simulink model "RBFNN_1221"  (R2018a)
settings: Solver=FixedStepAuto  StartTime=0.0  StopTime=inf  FixedStep=0.001  RelTol=1e-3  EnableMultiTasking=on
undefined symbols (not defined in the file): HIL, j, qc_get_step_size
libraries: dsparch4 x28, quarc_library x17, simulink x7, vrlib x1
(part 2 of 6)

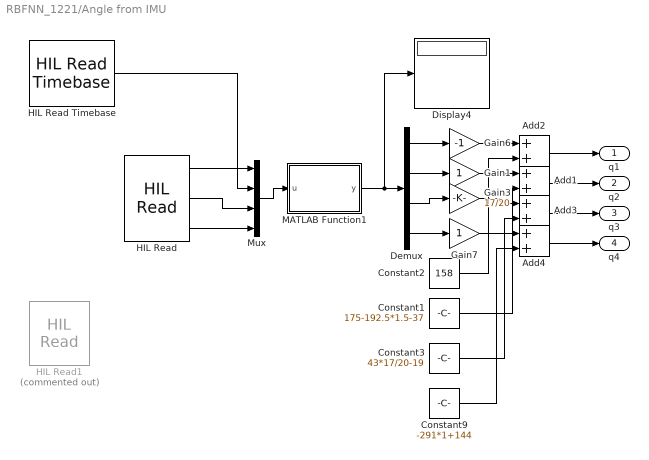
== system RBFNN_1221/Angle from IMU ==
  Add{1..4} (4 alike) : Sum
  Constant1 : Constant  Value=175-192.5*1.5-37
  Constant2 : Constant  Value=158
  Constant3 : Constant  Value=43*17/20-19
  Constant9 : Constant  Value=-291*1+144
  Demux : Demux
  Display4 : Display
  Gain1 : Gain
  Gain3 : Gain  Gain=17/20
  Gain6 : Gain  Gain=-1
  Gain7 : Gain
  HIL Read : quarc_library/Data Acquisition/Generic/Immediate I//O/HIL Read  object_name=HIL-1  analog_channels=[1 4 7]  encoder_channels=[]  digital_channels=[]  other_channels=[]  sample_time=qc_get_step_size  active=on  vector_output=off  data_type_mode=Inherit via back propagation  encoder_data_type=double  digital_data_type=boolean
  HIL Read Timebase : quarc_library/Data Acquisition/Generic/Timebases/HIL Read Timebase  object_name=HIL-2  clock=0  analog_channels=0  encoder_channels=[]  digital_channels=[]  other_channels=[]  samples_in_buffer=max(ceil(1/qc_get_step_size), 1)  active=on  vector_output=off  data_type_mode=Inherit via back propagation  encoder_data_type=double  digital_data_type=boolean
  HIL Read1 : quarc_library/Data Acquisition/Generic/Immediate I//O/HIL Read  Commented=on  object_name=HIL-2  analog_channels=[0]  encoder_channels=[]  digital_channels=[]  other_channels=[]  sample_time=qc_get_step_size  active=on  vector_output=off  data_type_mode=Inherit via back propagation  encoder_data_type=double  digital_data_type=boolean
  MATLAB Function1 : MATLAB Function  TreatAsAtomicUnit=on
  Mux : Mux
  q1 : Outport
  q2 : Outport  Port=2
  "q3 " : Outport  Port=3
  q4 : Outport  Port=4
  wires:
  Constant2/1 -> Add2/2
  Gain6/1 -> Add2/1
  Add2/1 -> q1/1
  Mux/1 -> MATLAB Function1/1(u)
  MATLAB Function1/1(y) -> Display4/1, Demux/1
  Demux/1 -> Gain6/1
  Gain3/1 -> Add3/1
  Gain7/1 -> Add4/1
  Constant3/1 -> Add3/2
  Constant9/1 -> Add4/2
  Add3/1 -> "q3 "/1
  Add4/1 -> q4/1
  HIL Read/1 -> Mux/1
  HIL Read/2 -> Mux/3
  HIL Read/3 -> Mux/4
  Demux/3 -> Gain3/1
  Demux/4 -> Gain7/1
  Demux/2 -> Gain1/1
  Gain1/1 -> Add1/1
  Constant1/1 -> Add1/2
  Add1/1 -> q2/1
  HIL Read Timebase/1 -> Mux/2

== system RBFNN_1221/Nan Switch ==
  control input : Inport
  angle signal : Inport  Port=2
  Constant4 : Constant  Value=0
  Mux : Mux
  Switch : Switch
  control : Outport
  wires:
  Switch/1 -> control/1
  control input/1 -> Switch/1
  angle signal/1 -> Switch/2
  Constant4/1 -> Mux/1, Mux/2, Mux/3, Mux/4
  Mux/1 -> Switch/3

== system RBFNN_1221/P1 ==
  Analog Filter Design1 : dsparch4/Analog Filter Design  method=Butterworth  filttype=Lowpass  N=2  Wlo=0.9  Whi=80  Rp=2  Rs=40
  Analog Filter Design2 : dsparch4/Analog Filter Design  method=Butterworth  filttype=Lowpass  N=2  Wlo=0.9  Whi=80  Rp=2  Rs=40
  HIL Read Analog : quarc_library/Data Acquisition/Generic/Immediate I//O/HIL Read Analog  object_name=HIL-1  channels=[2:3]  sample_time=qc_get_step_size  active=on  vector_output=off
  Manual Switch : ManualSwitch  CurrentSetting=0
  Manual Switch1 : ManualSwitch  CurrentSetting=0
  pin : Outport
  pout : Outport  Port=2
  wires:
  Manual Switch1/1 -> pout/1
  Manual Switch/1 -> pin/1
  HIL Read Analog/1 -> Analog Filter Design2/1, Manual Switch/1
  HIL Read Analog/2 -> Analog Filter Design1/1, Manual Switch1/1
  Analog Filter Design2/1 -> Manual Switch/2
  Analog Filter Design1/1 -> Manual Switch1/2

== system RBFNN_1221/P2 ==
  Analog Filter Design1 : dsparch4/Analog Filter Design  method=Butterworth  filttype=Lowpass  N=2  Wlo=0.9  Whi=80  Rp=2  Rs=40
  Analog Filter Design2 : dsparch4/Analog Filter Design  method=Butterworth  filttype=Lowpass  N=2  Wlo=0.9  Whi=80  Rp=2  Rs=40
  Demux : Demux  Outputs=2
  HIL Read Analog : quarc_library/Data Acquisition/Generic/Immediate I//O/HIL Read Analog  object_name=HIL-2  channels=[2:3]  sample_time=qc_get_step_size  active=on  vector_output=off
  Manual Switch : ManualSwitch
  Mux : Mux  Inputs=2
  Mux1 : Mux  Inputs=2
  pout : Outport
  pin : Outport  Port=2
  wires:
  HIL Read Analog/2 -> Analog Filter Design1/1
  HIL Read Analog/1 -> Analog Filter Design2/1
  Manual Switch/1 -> Demux/1
  Demux/1 -> pin/1
  Mux1/1 -> Manual Switch/2
  Mux/1 -> Manual Switch/1
  Analog Filter Design1/1 -> Mux1/1, Mux/2
  Demux/2 -> pout/1
  Analog Filter Design2/1 -> Mux1/2, Mux/1

== system RBFNN_1221/P3 ==
  Analog Filter Design1 : dsparch4/Analog Filter Design  method=Butterworth  filttype=Lowpass  N=2  Wlo=0.9  Whi=80  Rp=2  Rs=40
  Analog Filter Design2 : dsparch4/Analog Filter Design  method=Butterworth  filttype=Lowpass  N=2  Wlo=0.9  Whi=80  Rp=2  Rs=40
  HIL Read Analog : quarc_library/Data Acquisition/Generic/Immediate I//O/HIL Read Analog  object_name=HIL-1  channels=[5:6]  sample_time=qc_get_step_size  active=on  vector_output=off
  Scope : Scope  NumInputPorts=2
  pin : Outport
  pout : Outport  Port=2
  wires:
  Analog Filter Design1/1 -> pout/1
  Analog Filter Design2/1 -> pin/1
  HIL Read Analog/2 -> Scope/2, Analog Filter Design1/1
  HIL Read Analog/1 -> Scope/1, Analog Filter Design2/1

== system RBFNN_1221/P4 ==
  Analog Filter Design1 : dsparch4/Analog Filter Design  method=Butterworth  filttype=Lowpass  N=2  Wlo=0.9  Whi=80  Rp=2  Rs=40
  Analog Filter Design2 : dsparch4/Analog Filter Design  method=Butterworth  filttype=Lowpass  N=2  Wlo=0.9  Whi=80  Rp=2  Rs=40
  Demux : Demux  Outputs=2
  HIL Read Analog : quarc_library/Data Acquisition/Generic/Immediate I//O/HIL Read Analog  object_name=HIL-2  channels=[6:7]  sample_time=qc_get_step_size  active=on  vector_output=off
  Manual Switch : ManualSwitch
  Mux : Mux  Inputs=2
  Mux1 : Mux  Inputs=2
  pin : Outport
  pout : Outport  Port=2
  wires:
  HIL Read Analog/2 -> Analog Filter Design1/1
  HIL Read Analog/1 -> Analog Filter Design2/1
  Analog Filter Design2/1 -> Mux1/2, Mux/1
  Analog Filter Design1/1 -> Mux1/1, Mux/2
  Mux/1 -> Manual Switch/1
  Manual Switch/1 -> Demux/1
  Demux/1 -> pin/1
  Demux/2 -> pout/1
  Mux1/1 -> Manual Switch/2

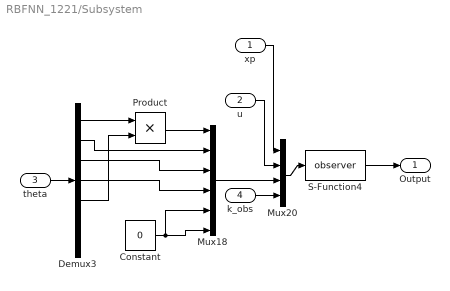
== system RBFNN_1221/Subsystem ==
  xp : Inport
  u : Inport  Port=2
  theta : Inport  Port=3
  k_obs : Inport  Port=4
  Constant : Constant  Value=0
  Demux3 : Demux  Outputs=7
  Mux18 : Mux  Inputs=6
  Mux20 : Mux
  Product : Product
  S-Function4 : S-Function  FunctionName=observer  SFunctionDeploymentMode=off  EnableBusSupport=off
  Output : Outport
  wires:
  theta/1 -> Demux3/1
  Demux3/1 -> Product/1
  Demux3/3 -> Mux18/3
  Mux18/1 -> Mux20/3
  Demux3/4 -> Mux18/4
  Demux3/5 -> Product/2
  Product/1 -> Mux18/1
  Mux20/1 -> S-Function4/1
  Demux3/2 -> Mux18/2
  k_obs/1 -> Mux20/4
  Constant/1 -> Mux18/5, Mux18/6
  S-Function4/1 -> Output/1
  u/1 -> Mux20/2
  xp/1 -> Mux20/1

== system RBFNN_1221/Subsystem1 ==
  xd : Inport
  xr : Inport  Port=2
  Sum : Sum  Inputs=+-
  qr : Outport
  e : Outport  Port=2
  wires:
  xr/1 -> Sum/2, qr/1
  xd/1 -> Sum/1
  Sum/1 -> e/1

== system RBFNN_1221/Subsystem2 ==
  xd : Inport
  xr : Inport  Port=2
  Sum : Sum  Inputs=+-
  qr : Outport
  e : Outport  Port=2
  wires:
  xr/1 -> Sum/2, qr/1
  xd/1 -> Sum/1
  Sum/1 -> e/1

== system RBFNN_1221/Subsystem3 ==
  xd : Inport
  xr : Inport  Port=2
  Sum : Sum  Inputs=+-
  qr : Outport
  e : Outport  Port=2
  wires:
  xr/1 -> Sum/2, qr/1
  xd/1 -> Sum/1
  Sum/1 -> e/1

== system RBFNN_1221/Subsystem4 ==
  xp : Inport
  u : Inport  Port=2
  theta : Inport  Port=3
  k_obs : Inport  Port=4
  Constant : Constant  Value=0
  Demux3 : Demux  Outputs=7
  Mux18 : Mux  Inputs=6
  Mux20 : Mux
  Product : Product
  S-Function4 : S-Function  FunctionName=observer3  SFunctionDeploymentMode=off  EnableBusSupport=off
  Output : Outport
  wires:
  theta/1 -> Demux3/1
  Demux3/1 -> Product/1
  Demux3/3 -> Mux18/3
  Mux18/1 -> Mux20/3
  Demux3/4 -> Mux18/4
  Demux3/5 -> Product/2
  Product/1 -> Mux18/1
  Mux20/1 -> S-Function4/1
  Demux3/2 -> Mux18/2
  k_obs/1 -> Mux20/4
  Constant/1 -> Mux18/5, Mux18/6
  S-Function4/1 -> Output/1
  u/1 -> Mux20/2
  xp/1 -> Mux20/1

== system RBFNN_1221/Subsystem5 ==
  xp : Inport
  u : Inport  Port=2
  theta : Inport  Port=3
  k_obs : Inport  Port=4
  Constant : Constant  Value=0
  Demux3 : Demux  Outputs=7
  Mux18 : Mux  Inputs=6
  Mux20 : Mux
  Product : Product
  S-Function4 : S-Function  FunctionName=observer2  SFunctionDeploymentMode=off  EnableBusSupport=off
  Output : Outport
  wires:
  theta/1 -> Demux3/1
  Demux3/1 -> Product/1
  Demux3/3 -> Mux18/3
  Mux18/1 -> Mux20/3
  Demux3/4 -> Mux18/4
  Demux3/5 -> Product/2
  Product/1 -> Mux18/1
  Mux20/1 -> S-Function4/1
  Demux3/2 -> Mux18/2
  k_obs/1 -> Mux20/4
  Constant/1 -> Mux18/5, Mux18/6
  S-Function4/1 -> Output/1
  u/1 -> Mux20/2
  xp/1 -> Mux20/1

== system RBFNN_1221/Subsystem6 ==
  xd : Inport
  xr : Inport  Port=2
  Sum : Sum  Inputs=+-
  qr : Outport
  e : Outport  Port=2
  wires:
  xr/1 -> Sum/2, qr/1
  xd/1 -> Sum/1
  Sum/1 -> e/1

== system RBFNN_1221/Subsystem7 ==
  xp : Inport
  u : Inport  Port=2
  theta : Inport  Port=3
  k_obs : Inport  Port=4
  Constant : Constant  Value=0
  Demux3 : Demux  Outputs=7
  Mux18 : Mux  Inputs=6
  Mux20 : Mux
  Product : Product
  S-Function4 : S-Function  FunctionName=observer4  SFunctionDeploymentMode=off  EnableBusSupport=off
  Output : Outport
  wires:
  theta/1 -> Demux3/1
  Demux3/1 -> Product/1
  Demux3/3 -> Mux18/3
  Mux18/1 -> Mux20/3
  Demux3/4 -> Mux18/4
  Demux3/5 -> Product/2
  Product/1 -> Mux18/1
  Mux20/1 -> S-Function4/1
  Demux3/2 -> Mux18/2
  k_obs/1 -> Mux20/4
  Constant/1 -> Mux18/5, Mux18/6
  S-Function4/1 -> Output/1
  u/1 -> Mux20/2
  xp/1 -> Mux20/1

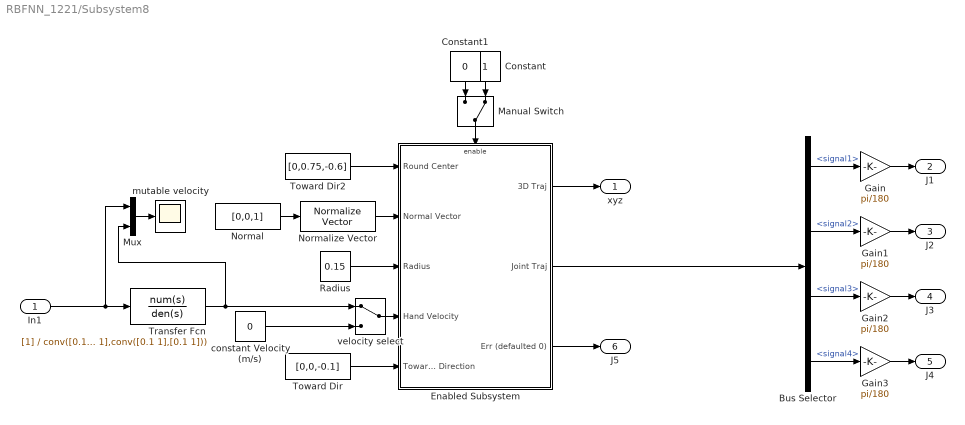
== system RBFNN_1221/Subsystem8 ==
  In1 : Inport
  Bus Selector : BusSelector  OutputSignals=signal1,signal2,signal3,signal4
  Constant : Constant
  Constant1 : Constant  Value=0
  Enabled Subsystem : Subsystem  TreatAsAtomicUnit=on
  Gain{,1..3} (4 alike) : Gain  Gain=pi/180
  Manual Switch : ManualSwitch  CurrentSetting=0
  Mux : Mux  Inputs=2
  Normal : Constant  Value=[0,0,1]
  Normalize Vector : vrlib/Utilities/Normalize Vector  maxzero=0
      settings: SourceProductName=Simulink
  Radius : Constant  Value=0.15
  Toward Dir : Constant  Value=[0,0,-0.1]
  Toward Dir2 : Constant  Value=[0,0.75,-0.6]
  Transfer Fcn : TransferFcn  Denominator=conv([0.1 1],conv([0.1 1],[0.1 1]))
  constant Velocity (m/s) : Constant  Value=0
  mutable velocity : Scope
  velocity select : ManualSwitch
  xyz : Outport
  J1 : Outport  Port=2
  J2 : Outport  Port=3
  J3 : Outport  Port=4
  J4 : Outport  Port=5
  J5 : Outport  Port=6
  wires:
  Toward Dir2/1 -> Enabled Subsystem/1(Round Center)
  In1/1 -> Mux/1, Transfer Fcn/1
  Normal/1 -> Normalize Vector/1
  Normalize Vector/1 -> Enabled Subsystem/2(Normal Vector)
  Enabled Subsystem/3(Err (defaulted 0)) -> J5/1
  Enabled Subsystem/2(Joint Traj) -> Bus Selector/1
  Manual Switch/1 -> Enabled Subsystem/Enable
  Constant1/1 -> Manual Switch/1
  Toward Dir/1 -> Enabled Subsystem/5(Toward Direction)
  Radius/1 -> Enabled Subsystem/3(Radius)
  Constant/1 -> Manual Switch/2
  Transfer Fcn/1 -> Mux/2, velocity select/1
  Mux/1 -> mutable velocity/1
  constant Velocity (m/s)/1 -> velocity select/2
  velocity select/1 -> Enabled Subsystem/4(Hand Velocity)
  Bus Selector/4 -> Gain3/1  "<signal4>"
  Bus Selector/3 -> Gain2/1  "<signal3>"
  Bus Selector/2 -> Gain1/1  "<signal2>"
  Enabled Subsystem/1(3D Traj) -> xyz/1
  Bus Selector/1 -> Gain/1  "<signal1>"
  Gain3/1 -> J4/1
  Gain2/1 -> J3/1
  Gain1/1 -> J2/1
  Gain/1 -> J1/1

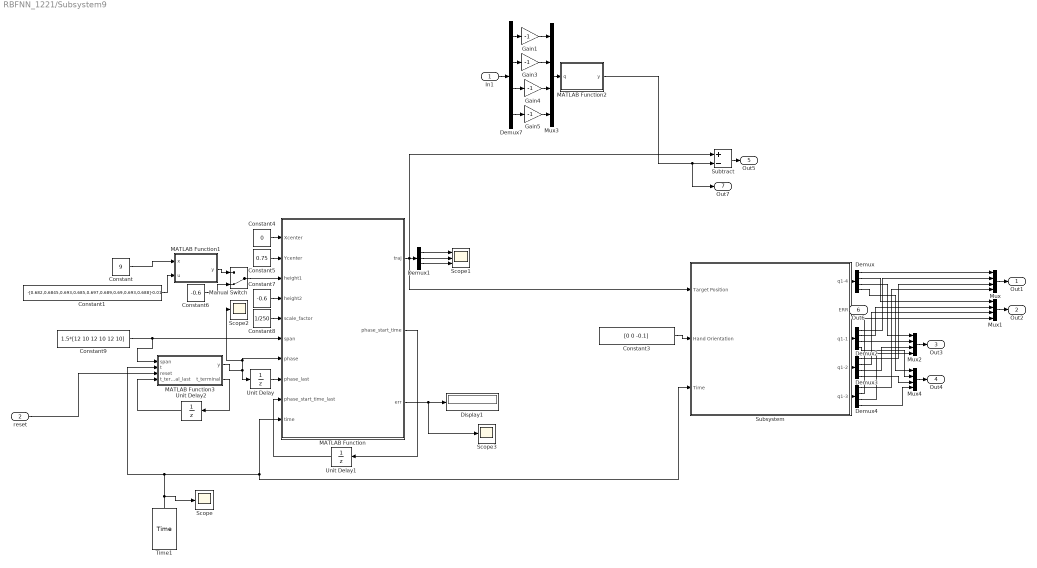
== system RBFNN_1221/Subsystem9 ==
  In1 : Inport
  reset : Inport  Port=2
  Constant : Constant  Value=9
  Constant1 : Constant  Value=-[0.682,0.6845,0.693,0.685,0.697,0.689,0.69,0.693,0.688]-0.01
  Constant3 : Constant  Value=[0 0 -0.1]
  Constant4 : Constant  Value=0
  Constant5 : Constant  Value=0.75
  Constant6 : Constant  Value=-0.6
  Constant7 : Constant  Value=-0.6
  Constant8 : Constant  Value=1/250
  Constant9 : Constant  Value=1.5*[12 10 12 10 12 10]
  Demux{,2..4,7} (5 alike) : Demux
  Demux1 : Demux  Outputs=3
  Display1 : Display
  Gain{1,3..5} (4 alike) : Gain  Gain=-1
  MATLAB Function : MATLAB Function  TreatAsAtomicUnit=on
  MATLAB Function1 : MATLAB Function  TreatAsAtomicUnit=on
  MATLAB Function2 : MATLAB Function  TreatAsAtomicUnit=on
  MATLAB Function3 : MATLAB Function  TreatAsAtomicUnit=on
  Manual Switch : ManualSwitch  CurrentSetting=0
  Mux{,1..4} (5 alike) : Mux
  Scope : Scope
  Scope1 : Scope  NumInputPorts=3
  Scope2 : Scope
  Scope3 : Scope
  Subsystem : Subsystem
  Subtract : Sum  Inputs=+-
  Time1 : quarc_library/Sources/Time/Time  time_source=Wall clock  sample_time=qc_get_step_size
  Unit Delay : UnitDelay  SampleTime=-1
  Unit Delay1 : UnitDelay  SampleTime=-1
  Unit Delay2 : UnitDelay  SampleTime=-1
  Out1 : Outport
  Out2 : Outport  Port=2
  Out3 : Outport  Port=3
  Out4 : Outport  Port=4
  Out5 : Outport  Port=5
  Out6 : Outport  Port=6
  Out7 : Outport  Port=7
  wires:
  Unit Delay/1 -> MATLAB Function/8(phase_last)
  MATLAB Function/1(traj) -> Subsystem/1(Target Position), Subtract/1, Demux1/1
  MATLAB Function/3(err) -> Scope3/1, Display1/1
  Constant3/1 -> Subsystem/2(Hand Orientation)
  Time1/1 -> Scope/1, MATLAB Function3/2(t), MATLAB Function/10(time), Subsystem/3(Time)
  MATLAB Function3/1(y) -> Unit Delay/1, MATLAB Function/7(phase), Scope2/1
  Constant9/1 -> MATLAB Function3/1(span), MATLAB Function/6(span)
  MATLAB Function/2(phase_start_time) -> Unit Delay1/1
  Constant5/1 -> MATLAB Function/2(Ycenter)
  Constant4/1 -> MATLAB Function/1(Xcenter)
  Demux1/3 -> Scope1/3
  Constant7/1 -> MATLAB Function/4(height2)
  Constant8/1 -> MATLAB Function/5(scale_factor)
  Demux1/1 -> Scope1/1
  Demux1/2 -> Scope1/2
  Unit Delay1/1 -> MATLAB Function/9(phase_start_time_last)
  Demux7/4 -> Gain5/1
  Gain4/1 -> Mux3/3
  Demux7/3 -> Gain4/1
  Demux7/2 -> Gain3/1
  Gain3/1 -> Mux3/2
  Gain5/1 -> Mux3/4
  In1/1 -> Demux7/1
  Mux3/1 -> MATLAB Function2/1(q)
  Subtract/1 -> Out5/1
  Subsystem/2(ERR) -> Out6/1
  Subsystem/1(q1-4) -> Demux/1
  Subsystem/3(q1-1) -> Demux2/1
  Subsystem/4(q1-2) -> Demux3/1
  Subsystem/5(q1-3) -> Demux4/1
  Demux/1 -> Mux/1
  Demux2/1 -> Mux/2
  Demux3/1 -> Mux/3
  Demux4/1 -> Mux/4
  Mux/1 -> Out1/1
  Demux/2 -> Mux1/1
  Demux2/2 -> Mux1/2
  Demux3/2 -> Mux1/3
  Demux4/2 -> Mux1/4
  Demux/3 -> Mux2/1
  Demux2/3 -> Mux2/2
  Demux3/3 -> Mux2/3
  Demux4/3 -> Mux2/4
  Demux/4 -> Mux4/1
  Demux2/4 -> Mux4/2
  Demux3/4 -> Mux4/3
  Demux4/4 -> Mux4/4
  Mux1/1 -> Out2/1
  Mux2/1 -> Out3/1
  Mux4/1 -> Out4/1
  reset/1 -> MATLAB Function3/3(reset)
  MATLAB Function3/2(t_terminal) -> Unit Delay2/1
  Unit Delay2/1 -> MATLAB Function3/4(t_terminal_last)
  Demux7/1 -> Gain1/1
  Gain1/1 -> Mux3/1
  MATLAB Function2/1(y) -> Out7/1, Subtract/2
  Constant1/1 -> MATLAB Function1/2(u)
  Manual Switch/1 -> MATLAB Function/3(height1)
  Constant6/1 -> Manual Switch/2
  MATLAB Function1/1(y) -> Manual Switch/1
  Constant/1 -> MATLAB Function1/1(x)

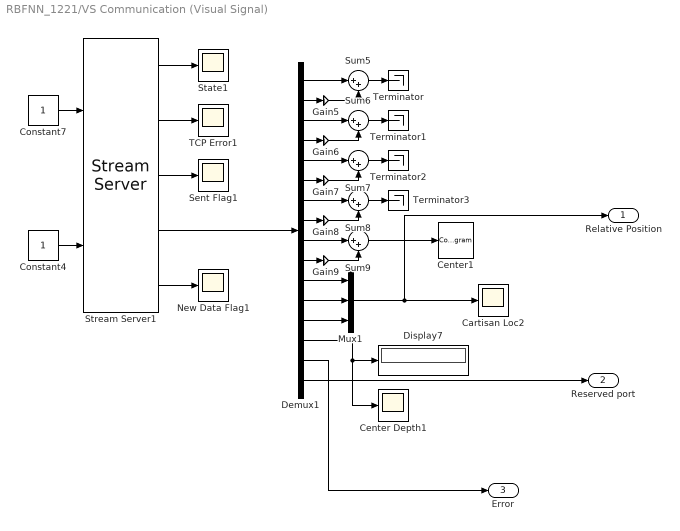
== system RBFNN_1221/VS Communication (Visual Signal) ==
  Cartisan Loc2 : Scope
  Center Depth1 : Scope
  Center1 : ConstellationDiagram
  Constant4 : Constant
  Constant7 : Constant
  Demux1 : Demux  Outputs=16
  Display7 : Display
  Gain{5..9} (5 alike) : Gain  Gain=j
  Mux1 : Mux  Inputs=3
  New Data Flag1 : Scope
  Sent Flag1 : Scope
  State1 : Scope
  Stream Server1 : quarc_library/Communications/Basic/Stream Server  uri_source=Specify via dialog (do not evaluate)  uri=tcpip://localhost:1804  apply_uri_to_all_configs=on  send_buffer_size=1460  receive_buffer_size=1460  byte_order=little endian (Intel - LSB first)  optimization=Minimum latency  send_options=Send most recent data  receive_options=Receive most recent data  default_value=[0;0;0;0;0;0;0;0;0;0;0;0;0;0;0;0]  sample_time=qc_get_step_size  active=off  implementation=Use blocking I/O in a separate thread  send_fifo_size=1000  receive_fifo_size=1000  send_priority=0  receive_priority=0  send_dimensions=off  receive_dimensions=off  max_dimensions=-1  data_type=double  type_expr=BusObject
      settings: AttributesFormatString="\"tcpip://localhost:1804\""
  Sum{5..9} (5 alike) : Sum  Inputs=|++
  TCP Error1 : Scope
  Terminator{,1..3} (4 alike) : Terminator
  Relative Position : Outport
  Reserved port : Outport  Port=2
  Error : Outport  Port=3
  wires:
  Demux1/14 -> Display7/1, Center Depth1/1
  Demux1/10 -> Gain9/1
  Demux1/5 -> Sum7/1
  Sum8/1 -> Terminator3/1
  Gain9/1 -> Sum9/2
  Mux1/1 -> Relative Position/1, Cartisan Loc2/1
  Gain8/1 -> Sum8/2
  Gain6/1 -> Sum6/2
  Demux1/3 -> Sum6/1
  Demux1/13 -> Mux1/3
  Stream Server1/2 -> TCP Error1/1
  Sum9/1 -> Center1/1
  Demux1/8 -> Gain8/1
  Stream Server1/3 -> Sent Flag1/1
  Demux1/15 -> Error/1
  Demux1/4 -> Gain6/1
  Stream Server1/5 -> New Data Flag1/1
  Demux1/6 -> Gain7/1
  Demux1/12 -> Mux1/2
  Sum6/1 -> Terminator1/1
  Constant4/1 -> Stream Server1/2
  Demux1/9 -> Sum9/1
  Gain7/1 -> Sum7/2
  Constant7/1 -> Stream Server1/1
  Demux1/2 -> Gain5/1
  Demux1/11 -> Mux1/1
  Demux1/1 -> Sum5/1
  Sum7/1 -> Terminator2/1
  Stream Server1/4 -> Demux1/1
  Stream Server1/1 -> State1/1
  Demux1/7 -> Sum8/1
  Gain5/1 -> Sum5/2
  Sum5/1 -> Terminator/1
  Demux1/16 -> Reserved port/1

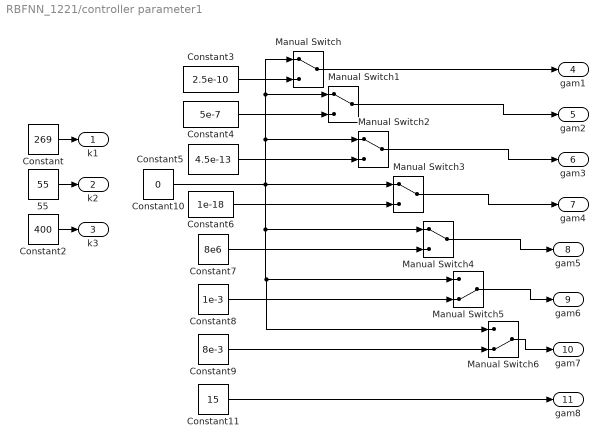
== system RBFNN_1221/controller parameter1 ==
  55 : Constant  Value=55
  Constant : Constant  Value=269
  Constant10 : Constant  Value=0
  Constant11 : Constant  Value=15
  Constant2 : Constant  Value=400
  Constant3 : Constant  Value=2.5e-10
  Constant4 : Constant  Value=5e-7
  Constant5 : Constant  Value=4.5e-13
  Constant6 : Constant  Value=1e-18
  Constant7 : Constant  Value=8e6
  Constant8 : Constant  Value=1e-3
  Constant9 : Constant  Value=8e-3
  Manual Switch{,1..4} (5 alike) : ManualSwitch
  Manual Switch5 : ManualSwitch  CurrentSetting=0
  Manual Switch6 : ManualSwitch  CurrentSetting=0
  k1 : Outport
  k2 : Outport  Port=2
  k3 : Outport  Port=3
  gam1 : Outport  Port=4
  gam2 : Outport  Port=5
  gam3 : Outport  Port=6
  gam4 : Outport  Port=7
  gam5 : Outport  Port=8
  gam6 : Outport  Port=9
  gam7 : Outport  Port=10
  gam8 : Outport  Port=11
  wires:
  Constant/1 -> k1/1
  55/1 -> k2/1
  Constant2/1 -> k3/1
  Manual Switch1/1 -> gam2/1
  Constant4/1 -> Manual Switch1/2
  Manual Switch/1 -> gam1/1
  Constant3/1 -> Manual Switch/2
  Constant10/1 -> Manual Switch/1, Manual Switch1/1, Manual Switch2/1, Manual Switch6/1, Manual Switch5/1, Manual Switch4/1, Manual Switch3/1
  Manual Switch2/1 -> gam3/1
  Constant5/1 -> Manual Switch2/2
  Manual Switch3/1 -> gam4/1
  Constant6/1 -> Manual Switch3/2
  Manual Switch4/1 -> gam5/1
  Constant7/1 -> Manual Switch4/2
  Manual Switch5/1 -> gam6/1
  Constant8/1 -> Manual Switch5/2
  Manual Switch6/1 -> gam7/1
  Constant9/1 -> Manual Switch6/2
  Constant11/1 -> gam8/1

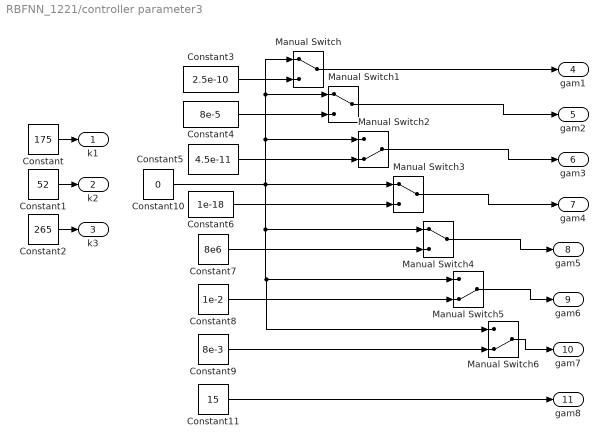
== system RBFNN_1221/controller parameter3 ==
  Constant : Constant  Value=175
  Constant1 : Constant  Value=52
  Constant10 : Constant  Value=0
  Constant11 : Constant  Value=15
  Constant2 : Constant  Value=265
  Constant3 : Constant  Value=2.5e-10
  Constant4 : Constant  Value=8e-5
  Constant5 : Constant  Value=4.5e-11
  Constant6 : Constant  Value=1e-18
  Constant7 : Constant  Value=8e6
  Constant8 : Constant  Value=1e-2
  Constant9 : Constant  Value=8e-3
  Manual Switch{,1,3..4} (4 alike) : ManualSwitch
  Manual Switch2 : ManualSwitch  CurrentSetting=0
  Manual Switch5 : ManualSwitch  CurrentSetting=0
  Manual Switch6 : ManualSwitch  CurrentSetting=0
  k1 : Outport
  k2 : Outport  Port=2
  k3 : Outport  Port=3
  gam1 : Outport  Port=4
  gam2 : Outport  Port=5
  gam3 : Outport  Port=6
  gam4 : Outport  Port=7
  gam5 : Outport  Port=8
  gam6 : Outport  Port=9
  gam7 : Outport  Port=10
  gam8 : Outport  Port=11
  wires:
  Constant/1 -> k1/1
  Constant1/1 -> k2/1
  Constant2/1 -> k3/1
  Manual Switch1/1 -> gam2/1
  Constant4/1 -> Manual Switch1/2
  Manual Switch/1 -> gam1/1
  Constant3/1 -> Manual Switch/2
  Constant10/1 -> Manual Switch/1, Manual Switch1/1, Manual Switch2/1, Manual Switch6/1, Manual Switch5/1, Manual Switch4/1, Manual Switch3/1
  Manual Switch2/1 -> gam3/1
  Constant5/1 -> Manual Switch2/2
  Manual Switch3/1 -> gam4/1
  Constant6/1 -> Manual Switch3/2
  Manual Switch4/1 -> gam5/1
  Constant7/1 -> Manual Switch4/2
  Manual Switch5/1 -> gam6/1
  Constant8/1 -> Manual Switch5/2
  Manual Switch6/1 -> gam7/1
  Constant9/1 -> Manual Switch6/2
  Constant11/1 -> gam8/1

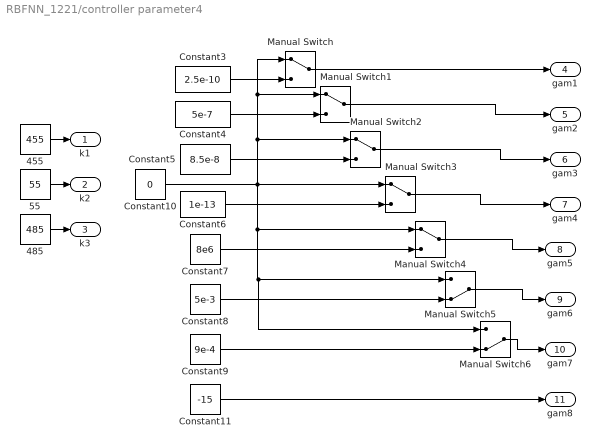
== system RBFNN_1221/controller parameter4 ==
  " 455" : Constant  Value=455
  485 : Constant  Value=485
  55 : Constant  Value=55
  Constant10 : Constant  Value=0
  Constant11 : Constant  Value=-15
  Constant3 : Constant  Value=2.5e-10
  Constant4 : Constant  Value=5e-7
  Constant5 : Constant  Value=8.5e-8
  Constant6 : Constant  Value=1e-13
  Constant7 : Constant  Value=8e6
  Constant8 : Constant  Value=5e-3
  Constant9 : Constant  Value=9e-4
  Manual Switch{,1..4} (5 alike) : ManualSwitch
  Manual Switch5 : ManualSwitch  CurrentSetting=0
  Manual Switch6 : ManualSwitch  CurrentSetting=0
  k1 : Outport
  k2 : Outport  Port=2
  k3 : Outport  Port=3
  gam1 : Outport  Port=4
  gam2 : Outport  Port=5
  gam3 : Outport  Port=6
  gam4 : Outport  Port=7
  gam5 : Outport  Port=8
  gam6 : Outport  Port=9
  gam7 : Outport  Port=10
  gam8 : Outport  Port=11
  wires:
  " 455"/1 -> k1/1
  55/1 -> k2/1
  485/1 -> k3/1
  Manual Switch1/1 -> gam2/1
  Constant4/1 -> Manual Switch1/2
  Manual Switch/1 -> gam1/1
  Constant3/1 -> Manual Switch/2
  Constant10/1 -> Manual Switch/1, Manual Switch1/1, Manual Switch2/1, Manual Switch6/1, Manual Switch5/1, Manual Switch4/1, Manual Switch3/1
  Manual Switch2/1 -> gam3/1
  Constant5/1 -> Manual Switch2/2
  Manual Switch3/1 -> gam4/1
  Constant6/1 -> Manual Switch3/2
  Manual Switch4/1 -> gam5/1
  Constant7/1 -> Manual Switch4/2
  Manual Switch5/1 -> gam6/1
  Constant8/1 -> Manual Switch5/2
  Manual Switch6/1 -> gam7/1
  Constant9/1 -> Manual Switch6/2
  Constant11/1 -> gam8/1

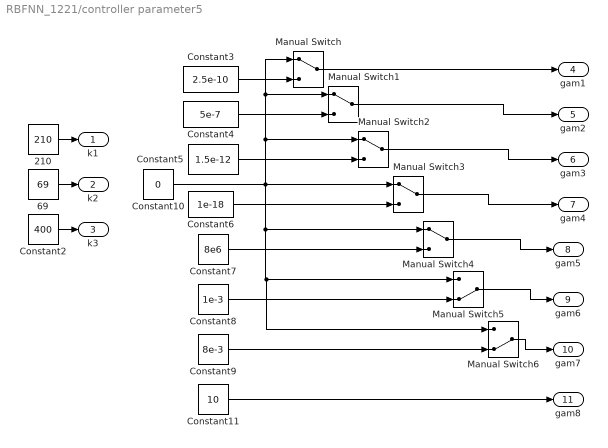
== system RBFNN_1221/controller parameter5 ==
  210 : Constant  Value=210
  69 : Constant  Value=69
  Constant10 : Constant  Value=0
  Constant11 : Constant  Value=10
  Constant2 : Constant  Value=400
  Constant3 : Constant  Value=2.5e-10
  Constant4 : Constant  Value=5e-7
  Constant5 : Constant  Value=1.5e-12
  Constant6 : Constant  Value=1e-18
  Constant7 : Constant  Value=8e6
  Constant8 : Constant  Value=1e-3
  Constant9 : Constant  Value=8e-3
  Manual Switch{,1..4} (5 alike) : ManualSwitch
  Manual Switch5 : ManualSwitch  CurrentSetting=0
  Manual Switch6 : ManualSwitch  CurrentSetting=0
  k1 : Outport
  k2 : Outport  Port=2
  k3 : Outport  Port=3
  gam1 : Outport  Port=4
  gam2 : Outport  Port=5
  gam3 : Outport  Port=6
  gam4 : Outport  Port=7
  gam5 : Outport  Port=8
  gam6 : Outport  Port=9
  gam7 : Outport  Port=10
  gam8 : Outport  Port=11
  wires:
  210/1 -> k1/1
  69/1 -> k2/1
  Constant2/1 -> k3/1
  Manual Switch1/1 -> gam2/1
  Constant4/1 -> Manual Switch1/2
  Manual Switch/1 -> gam1/1
  Constant3/1 -> Manual Switch/2
  Constant10/1 -> Manual Switch/1, Manual Switch1/1, Manual Switch2/1, Manual Switch6/1, Manual Switch5/1, Manual Switch4/1, Manual Switch3/1
  Manual Switch2/1 -> gam3/1
  Constant5/1 -> Manual Switch2/2
  Manual Switch3/1 -> gam4/1
  Constant6/1 -> Manual Switch3/2
  Manual Switch4/1 -> gam5/1
  Constant7/1 -> Manual Switch4/2
  Manual Switch5/1 -> gam6/1
  Constant8/1 -> Manual Switch5/2
  Manual Switch6/1 -> gam7/1
  Constant9/1 -> Manual Switch6/2
  Constant11/1 -> gam8/1

== system RBFNN_1221/pressure detect ==
  Analog Filter Design1 : dsparch4/Analog Filter Design  method=Butterworth  filttype=Lowpass  N=2  Wlo=0.9  Whi=80  Rp=2  Rs=40
  Analog Filter Design2 : dsparch4/Analog Filter Design  method=Butterworth  filttype=Lowpass  N=2  Wlo=0.9  Whi=80  Rp=2  Rs=40
  HIL Read Analog : quarc_library/Data Acquisition/Generic/Immediate I//O/HIL Read Analog  object_name=HIL-1  channels=[2:3]  sample_time=qc_get_step_size  active=on  vector_output=off
  Manual Switch : ManualSwitch  CurrentSetting=0
  Manual Switch1 : ManualSwitch  CurrentSetting=0
  pin : Outport
  pout : Outport  Port=2
  wires:
  Manual Switch1/1 -> pout/1
  Manual Switch/1 -> pin/1
  HIL Read Analog/1 -> Analog Filter Design2/1, Manual Switch/1
  HIL Read Analog/2 -> Analog Filter Design1/1, Manual Switch1/1
  Analog Filter Design2/1 -> Manual Switch/2
  Analog Filter Design1/1 -> Manual Switch1/2

== system RBFNN_1221/pressure detect1 ==
  Analog Filter Design1 : dsparch4/Analog Filter Design  method=Butterworth  filttype=Lowpass  N=2  Wlo=0.9  Whi=80  Rp=2  Rs=40
  Analog Filter Design2 : dsparch4/Analog Filter Design  method=Butterworth  filttype=Lowpass  N=2  Wlo=0.9  Whi=80  Rp=2  Rs=40
  HIL Read Analog : quarc_library/Data Acquisition/Generic/Immediate I//O/HIL Read Analog  object_name=HIL-1  channels=[5:6]  sample_time=qc_get_step_size  active=on  vector_output=off
  Scope : Scope  NumInputPorts=2
  pin : Outport
  pout : Outport  Port=2
  wires:
  Analog Filter Design1/1 -> pout/1
  Analog Filter Design2/1 -> pin/1
  HIL Read Analog/2 -> Scope/2, Analog Filter Design1/1
  HIL Read Analog/1 -> Scope/1, Analog Filter Design2/1

== system RBFNN_1221/pressure detect2 ==
  Analog Filter Design1 : dsparch4/Analog Filter Design  method=Butterworth  filttype=Lowpass  N=2  Wlo=0.9  Whi=80  Rp=2  Rs=40
  Analog Filter Design2 : dsparch4/Analog Filter Design  method=Butterworth  filttype=Lowpass  N=2  Wlo=0.9  Whi=80  Rp=2  Rs=40
  Demux : Demux  Outputs=2
  HIL Read Analog : quarc_library/Data Acquisition/Generic/Immediate I//O/HIL Read Analog  object_name=HIL-2  channels=[2:3]  sample_time=qc_get_step_size  active=on  vector_output=off
  Manual Switch : ManualSwitch
  Mux : Mux  Inputs=2
  Mux1 : Mux  Inputs=2
  pin : Outport
  pout : Outport  Port=2
  wires:
  HIL Read Analog/2 -> Analog Filter Design1/1
  HIL Read Analog/1 -> Analog Filter Design2/1
  Manual Switch/1 -> Demux/1
  Demux/1 -> pin/1
  Mux1/1 -> Manual Switch/2
  Mux/1 -> Manual Switch/1
  Analog Filter Design1/1 -> Mux1/1, Mux/2
  Demux/2 -> pout/1
  Analog Filter Design2/1 -> Mux1/2, Mux/1

== system RBFNN_1221/pressure detect3 ==
  Analog Filter Design1 : dsparch4/Analog Filter Design  method=Butterworth  filttype=Lowpass  N=2  Wlo=0.9  Whi=80  Rp=2  Rs=40
  Analog Filter Design2 : dsparch4/Analog Filter Design  method=Butterworth  filttype=Lowpass  N=2  Wlo=0.9  Whi=80  Rp=2  Rs=40
  Demux : Demux  Outputs=2
  HIL Read Analog : quarc_library/Data Acquisition/Generic/Immediate I//O/HIL Read Analog  object_name=HIL-2  channels=[6:7]  sample_time=qc_get_step_size  active=on  vector_output=off
  Manual Switch : ManualSwitch
  Mux : Mux  Inputs=2
  Mux1 : Mux  Inputs=2
  pin : Outport
  pout : Outport  Port=2
  wires:
  HIL Read Analog/2 -> Analog Filter Design1/1
  HIL Read Analog/1 -> Analog Filter Design2/1
  Analog Filter Design2/1 -> Mux1/2, Mux/1
  Analog Filter Design1/1 -> Mux1/1, Mux/2
  Mux/1 -> Manual Switch/1
  Manual Switch/1 -> Demux/1
  Demux/1 -> pin/1
  Demux/2 -> pout/1
  Mux1/1 -> Manual Switch/2

== system RBFNN_1221/velocity caculator ==
  xr : Inport
  Add : Sum  Inputs=+-
  Analog Filter Design : dsparch4/Analog Filter Design  method=Butterworth  filttype=Lowpass  N=2  Wlo=100  Whi=80  Rp=2  Rs=40
  Constant1 : Constant  Value=0.00125
  Data Store Memory : DataStoreMemory  DataStoreName=angle  ReadBeforeWriteMsg=warning  WriteAfterWriteMsg=warning  WriteAfterReadMsg=warning  ShowAdditionalParam=off
  Data Store Read : DataStoreRead  DataStoreName=angle
  Data Store Write : DataStoreWrite  DataStoreName=angle
  Delay : Delay  DelayLength=5
  Divide : Product  Inputs=*/
  dxr : Outport
  dxb : Outport  Port=2
  wires:
  Analog Filter Design/1 -> dxr/1
  xr/1 -> Add/1, Delay/1
  Data Store Read/1 -> Add/2
  Delay/1 -> Data Store Write/1
  Constant1/1 -> Divide/2
  Add/1 -> Divide/1
  Divide/1 -> dxb/1, Analog Filter Design/1

== system RBFNN_1221/velocity caculator1 ==
  xr : Inport
  Add : Sum  Inputs=+-
  Analog Filter Design : dsparch4/Analog Filter Design  method=Butterworth  filttype=Lowpass  N=2  Wlo=0.9  Whi=80  Rp=2  Rs=40
  Constant1 : Constant  Value=0.00125
  Data Store Memory : DataStoreMemory  DataStoreName=angle  ReadBeforeWriteMsg=warning  WriteAfterWriteMsg=warning  WriteAfterReadMsg=warning  ShowAdditionalParam=off
  Data Store Read : DataStoreRead  DataStoreName=angle
  Data Store Write : DataStoreWrite  DataStoreName=angle
  Delay : Delay  DelayLength=5
  Divide : Product  Inputs=*/
  dxr : Outport
  wires:
  Analog Filter Design/1 -> dxr/1
  xr/1 -> Add/1, Delay/1
  Data Store Read/1 -> Add/2
  Delay/1 -> Data Store Write/1
  Constant1/1 -> Divide/2
  Add/1 -> Divide/1
  Divide/1 -> Analog Filter Design/1

== system RBFNN_1221/velocity caculator2 ==
  xr : Inport
  Add : Sum  Inputs=+-
  Analog Filter Design : dsparch4/Analog Filter Design  method=Butterworth  filttype=Lowpass  N=2  Wlo=0.9  Whi=80  Rp=2  Rs=40
  Constant1 : Constant  Value=0.00125
  Data Store Memory : DataStoreMemory  DataStoreName=angle  ReadBeforeWriteMsg=warning  WriteAfterWriteMsg=warning  WriteAfterReadMsg=warning  ShowAdditionalParam=off
  Data Store Read : DataStoreRead  DataStoreName=angle
  Data Store Write : DataStoreWrite  DataStoreName=angle
  Delay : Delay  DelayLength=5
  Divide : Product  Inputs=*/
  dxr : Outport
  wires:
  Analog Filter Design/1 -> dxr/1
  xr/1 -> Add/1, Delay/1
  Data Store Read/1 -> Add/2
  Delay/1 -> Data Store Write/1
  Constant1/1 -> Divide/2
  Add/1 -> Divide/1
  Divide/1 -> Analog Filter Design/1

== system RBFNN_1221/velocity caculator3 ==
  xr : Inport
  Add : Sum  Inputs=+-
  Analog Filter Design : dsparch4/Analog Filter Design  method=Butterworth  filttype=Lowpass  N=2  Wlo=0.9  Whi=80  Rp=2  Rs=40
  Constant1 : Constant  Value=0.00125
  Data Store Memory : DataStoreMemory  DataStoreName=angle  ReadBeforeWriteMsg=warning  WriteAfterWriteMsg=warning  WriteAfterReadMsg=warning  ShowAdditionalParam=off
  Data Store Read : DataStoreRead  DataStoreName=angle
  Data Store Write : DataStoreWrite  DataStoreName=angle
  Delay : Delay  DelayLength=5
  Divide : Product  Inputs=*/
  dxr : Outport
  wires:
  Analog Filter Design/1 -> dxr/1
  xr/1 -> Add/1, Delay/1
  Data Store Read/1 -> Add/2
  Delay/1 -> Data Store Write/1
  Constant1/1 -> Divide/2
  Add/1 -> Divide/1
  Divide/1 -> Analog Filter Design/1

== system RBFNN_1221/velocity caculator4 ==
  xr : Inport
  Add : Sum  Inputs=+-
  Analog Filter Design : dsparch4/Analog Filter Design  method=Butterworth  filttype=Lowpass  N=2  Wlo=0.9  Whi=80  Rp=2  Rs=40
  Constant1 : Constant  Value=0.001
  Data Store Memory : DataStoreMemory  DataStoreName=angle  ReadBeforeWriteMsg=warning  WriteAfterWriteMsg=warning  WriteAfterReadMsg=warning  ShowAdditionalParam=off
  Data Store Read : DataStoreRead  DataStoreName=angle
  Data Store Write : DataStoreWrite  DataStoreName=angle
  Delay : Delay  DelayLength=1
  Divide : Product  Inputs=*/
  dxr : Outport
  wires:
  Divide/1 -> dxr/1
  xr/1 -> Delay/1, Add/1
  Data Store Read/1 -> Add/2
  Delay/1 -> Data Store Write/1
  Constant1/1 -> Divide/2
  Add/1 -> Divide/1

== system RBFNN_1221/velocity caculator5 ==
  xr : Inport
  Add : Sum  Inputs=+-
  Analog Filter Design : dsparch4/Analog Filter Design  method=Butterworth  filttype=Lowpass  N=2  Wlo=0.9  Whi=80  Rp=2  Rs=40
  Constant1 : Constant  Value=0.001
  Data Store Memory : DataStoreMemory  DataStoreName=angle  ReadBeforeWriteMsg=warning  WriteAfterWriteMsg=warning  WriteAfterReadMsg=warning  ShowAdditionalParam=off
  Data Store Read : DataStoreRead  DataStoreName=angle
  Data Store Write : DataStoreWrite  DataStoreName=angle
  Delay : Delay  DelayLength=1
  Divide : Product  Inputs=*/
  dxr : Outport
  wires:
  Analog Filter Design/1 -> dxr/1
  xr/1 -> Add/1, Delay/1
  Data Store Read/1 -> Add/2
  Delay/1 -> Data Store Write/1
  Constant1/1 -> Divide/2
  Add/1 -> Divide/1
  Divide/1 -> Analog Filter Design/1

== system RBFNN_1221/velocity caculator6 ==
  xr : Inport
  Add : Sum  Inputs=+-
  Analog Filter Design : dsparch4/Analog Filter Design  method=Butterworth  filttype=Lowpass  N=2  Wlo=0.9  Whi=80  Rp=2  Rs=40
  Constant1 : Constant  Value=0.001
  Data Store Memory : DataStoreMemory  DataStoreName=angle  ReadBeforeWriteMsg=warning  WriteAfterWriteMsg=warning  WriteAfterReadMsg=warning  ShowAdditionalParam=off
  Data Store Read : DataStoreRead  DataStoreName=angle
  Data Store Write : DataStoreWrite  DataStoreName=angle
  Delay : Delay  DelayLength=1
  Divide : Product  Inputs=*/
  dxr : Outport
  wires:
  Analog Filter Design/1 -> dxr/1
  xr/1 -> Add/1, Delay/1
  Data Store Read/1 -> Add/2
  Delay/1 -> Data Store Write/1
  Constant1/1 -> Divide/2
  Add/1 -> Divide/1
  Divide/1 -> Analog Filter Design/1

== system RBFNN_1221/velocity caculator7 ==
  xr : Inport
  Add : Sum  Inputs=+-
  Analog Filter Design : dsparch4/Analog Filter Design  method=Butterworth  filttype=Lowpass  N=2  Wlo=0.9  Whi=80  Rp=2  Rs=40
  Constant1 : Constant  Value=0.001
  Data Store Memory : DataStoreMemory  DataStoreName=angle  ReadBeforeWriteMsg=warning  WriteAfterWriteMsg=warning  WriteAfterReadMsg=warning  ShowAdditionalParam=off
  Data Store Read : DataStoreRead  DataStoreName=angle
  Data Store Write : DataStoreWrite  DataStoreName=angle
  Delay : Delay  DelayLength=1
  Divide : Product  Inputs=*/
  dxr : Outport
  wires:
  Analog Filter Design/1 -> dxr/1
  xr/1 -> Add/1, Delay/1
  Data Store Read/1 -> Add/2
  Delay/1 -> Data Store Write/1
  Constant1/1 -> Divide/2
  Add/1 -> Divide/1
  Divide/1 -> Analog Filter Design/1

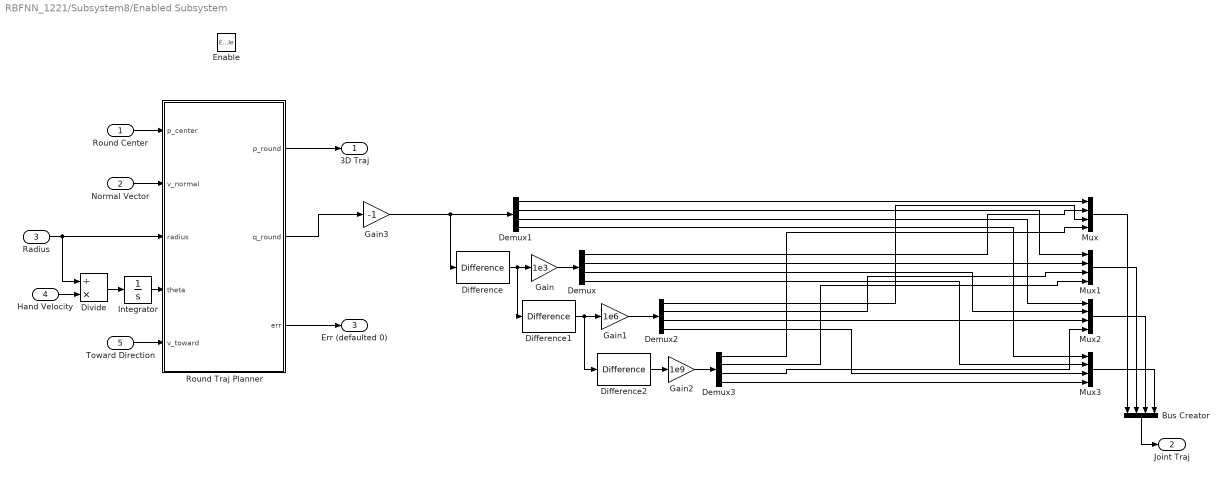
== system RBFNN_1221/Subsystem8/Enabled Subsystem ==
  Round Center : Inport
  Normal Vector : Inport  Port=2
  Radius : Inport  Port=3
  Hand Velocity : Inport  Port=4
  Toward Direction : Inport  Port=5
  Enable : EnablePort
  Bus Creator : BusCreator  Inputs=4
  Demux{,1..3} (4 alike) : Demux
  Difference : simulink/Discrete/Difference  ICPrevInput=0.0  OutMin=[]  OutMax=[]  OutDataType=fixdt(1, 16)  OutScaling=2^-10  DoSatur=off
  Difference1 : simulink/Discrete/Difference  ICPrevInput=0.0  OutMin=[]  OutMax=[]  OutDataType=fixdt(1, 16)  OutScaling=2^-10  DoSatur=off
  Difference2 : simulink/Discrete/Difference  ICPrevInput=0.0  OutMin=[]  OutMax=[]  OutDataType=fixdt(1, 16)  OutScaling=2^-10  DoSatur=off
  Divide : Product  Inputs=/*
  Gain : Gain  Gain=1e3
  Gain1 : Gain  Gain=1e6
  Gain2 : Gain  Gain=1e9
  Gain3 : Gain  Gain=-1
  Integrator : Integrator
  Mux{,1..3} (4 alike) : Mux
  Round Traj Planner : MATLAB Function  TreatAsAtomicUnit=on
  3D Traj : Outport  VectorParamsAs1DForOutWhenUnconnected=on
  Joint Traj : Outport  Port=2  VectorParamsAs1DForOutWhenUnconnected=on
  Err (defaulted 0) : Outport  Port=3  VectorParamsAs1DForOutWhenUnconnected=on
  wires:
  Normal Vector/1 -> Round Traj Planner/2(v_normal)
  Round Center/1 -> Round Traj Planner/1(p_center)
  Radius/1 -> Divide/1, Round Traj Planner/3(radius)
  Hand Velocity/1 -> Divide/2
  Divide/1 -> Integrator/1
  Integrator/1 -> Round Traj Planner/4(theta)
  Toward Direction/1 -> Round Traj Planner/5(v_toward)
  Round Traj Planner/3(err) -> Err (defaulted 0)/1
  Round Traj Planner/1(p_round) -> 3D Traj/1
  Demux1/4 -> Mux3/1
  Mux2/1 -> Bus Creator/3
  Demux2/1 -> Mux/3
  Demux/3 -> Mux2/2
  Demux3/3 -> Mux2/4
  Mux3/1 -> Bus Creator/4
  Gain2/1 -> Demux3/1
  Difference1/1 -> Gain1/1, Difference2/1
  Gain/1 -> Demux/1
  Demux/2 -> Mux1/2
  Demux1/2 -> Mux1/1
  Difference2/1 -> Gain2/1
  Demux2/2 -> Mux1/3
  Demux3/4 -> Mux3/4
  Demux/4 -> Mux3/2
  Demux3/2 -> Mux1/4
  Round Traj Planner/2(q_round) -> Gain3/1
  Demux/1 -> Mux/2
  Mux/1 -> Bus Creator/1
  Mux1/1 -> Bus Creator/2
  Demux2/3 -> Mux2/3
  Difference/1 -> Difference1/1, Gain/1
  Bus Creator/1 -> Joint Traj/1
  Demux1/3 -> Mux2/1
  Gain1/1 -> Demux2/1
  Demux3/1 -> Mux/4
  Demux2/4 -> Mux3/3
  Demux1/1 -> Mux/1
  Gain3/1 -> Demux1/1, Difference/1

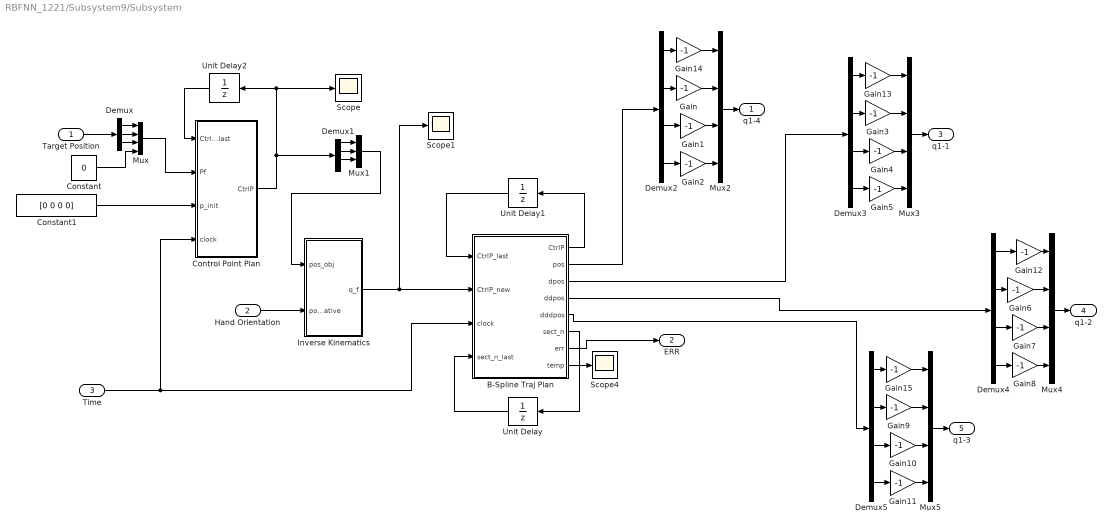
== system RBFNN_1221/Subsystem9/Subsystem ==
  Target Position : Inport
  Hand Orientation : Inport  Port=2
  Time : Inport  Port=3
  B-Spline Traj Plan : MATLAB Function  TreatAsAtomicUnit=on
  Constant : Constant  Value=0
  Constant1 : Constant  Value=[0 0 0 0]
  Control Point Plan : MATLAB Function  TreatAsAtomicUnit=on
  Demux : Demux  Outputs=3
  Demux{1..5} (5 alike) : Demux
  Gain{,1..15} (16 alike) : Gain  Gain=-1
  Inverse Kinematics : MATLAB Function  TreatAsAtomicUnit=on
  Mux{,2..5} (5 alike) : Mux
  Mux1 : Mux  Inputs=3
  Scope : Scope
  Scope1 : Scope
  Scope4 : Scope
  Unit Delay : UnitDelay  SampleTime=-1
  Unit Delay1 : UnitDelay  SampleTime=-1
  Unit Delay2 : UnitDelay  SampleTime=-1
  q1-4 : Outport  VectorParamsAs1DForOutWhenUnconnected=on
  ERR : Outport  Port=2  VectorParamsAs1DForOutWhenUnconnected=on
  q1-1 : Outport  Port=3  VectorParamsAs1DForOutWhenUnconnected=on
  q1-2 : Outport  Port=4  VectorParamsAs1DForOutWhenUnconnected=on
  q1-3 : Outport  Port=5  VectorParamsAs1DForOutWhenUnconnected=on
  wires:
  B-Spline Traj Plan/5(dddpos) -> Demux5/1
  Inverse Kinematics/1(q_f) -> Scope1/1, B-Spline Traj Plan/2(CtrlP_new)
  Time/1 -> Control Point Plan/4(clock), B-Spline Traj Plan/3(clock)
  B-Spline Traj Plan/3(dpos) -> Demux3/1
  Target Position/1 -> Demux/1
  B-Spline Traj Plan/1(CtrlP) -> Unit Delay1/1
  Unit Delay/1 -> B-Spline Traj Plan/4(sect_n_last)
  Unit Delay1/1 -> B-Spline Traj Plan/1(CtrlP_last)
  B-Spline Traj Plan/8(temp) -> Scope4/1
  B-Spline Traj Plan/6(sect_n) -> Unit Delay/1
  B-Spline Traj Plan/7(err) -> ERR/1
  Hand Orientation/1 -> Inverse Kinematics/2(pos_relative)
  Demux/1 -> Mux/1
  Demux/2 -> Mux/2
  Demux/3 -> Mux/3
  Constant/1 -> Mux/4
  Mux/1 -> Control Point Plan/2(Pf)
  Unit Delay2/1 -> Control Point Plan/1(CtrlP_last)
  Control Point Plan/1(CtrlP) -> Demux1/1, Scope/1, Unit Delay2/1
  Constant1/1 -> Control Point Plan/3(p_init)
  Demux1/1 -> Mux1/1
  Demux1/2 -> Mux1/2
  Demux1/3 -> Mux1/3
  Mux1/1 -> Inverse Kinematics/1(pos_obj)
  Demux2/2 -> Gain/1
  Gain/1 -> Mux2/2
  Demux2/3 -> Gain1/1
  Gain1/1 -> Mux2/3
  Demux2/4 -> Gain2/1
  Gain2/1 -> Mux2/4
  Mux2/1 -> q1-4/1
  B-Spline Traj Plan/2(pos) -> Demux2/1
  Gain4/1 -> Mux3/3
  Demux3/4 -> Gain5/1
  Demux3/2 -> Gain3/1
  Gain3/1 -> Mux3/2
  Mux3/1 -> q1-1/1
  Gain5/1 -> Mux3/4
  Demux3/3 -> Gain4/1
  Gain7/1 -> Mux4/3
  Demux4/4 -> Gain8/1
  Demux4/2 -> Gain6/1
  Gain6/1 -> Mux4/2
  Mux4/1 -> q1-2/1
  Gain8/1 -> Mux4/4
  Demux4/3 -> Gain7/1
  B-Spline Traj Plan/4(ddpos) -> Demux4/1
  Gain10/1 -> Mux5/3
  Demux5/4 -> Gain11/1
  Demux5/2 -> Gain9/1
  Gain9/1 -> Mux5/2
  Mux5/1 -> q1-3/1
  Gain11/1 -> Mux5/4
  Demux5/3 -> Gain10/1
  Demux4/1 -> Gain12/1
  Gain12/1 -> Mux4/1
  Demux3/1 -> Gain13/1
  Gain13/1 -> Mux3/1
  Demux2/1 -> Gain14/1
  Gain14/1 -> Mux2/1
  Demux5/1 -> Gain15/1
  Gain15/1 -> Mux5/1

== matlab function RBFNN_1221/Obs Para Generator1 ==
  data: a input; gain input; k_obs output; th input
function k_obs = fcn(a, gain, th)

if a <= th
    b = 22.5*a-37.5;
else
    b = 31.16*a - 68.8; % a>=2.5
end
k_obs  = ([1 1/a 1/b] .* gain.^[1 2 3])';

== matlab function RBFNN_1221/limit_u ==
  data: u input; y output
function y = fcn(u)
y=u;
if u>10
    y=10;
end
if u<-10
    y=-10;
end
end

== matlab function RBFNN_1221/MATLAB Function ==
  data: bias input; out output; xv input
function out = fcn(bias,xv)
out = xv;
if xv > 0
    out = xv + bias;
end
if xv < 0
    out = xv - bias;
end
end

== matlab function RBFNN_1221/Obs Para Generator2 ==
  data: a input; gain input; k_obs output; th input
function k_obs = fcn(a, gain, th)

if a <= th
    b = 22.5*a-37.5;
else
    b = 31.16*a - 68.8; % a>=2.5
end
k_obs  = ([1 1/a 1/b] .* gain.^[1 2 3])';

== matlab function RBFNN_1221/MATLAB Function10 ==
  data: p_end input; s output; v_max input; a_max input; ts input; t input; v output; a output; j output
function [s, v, a, j] = fcn(p_end, v_max, a_max, ts, t)
y=[0,0,0,0];

v_M=v_max;
a_M=a_max;

j_M	  = a_M*20.0;  % Max jerk (the rate of acceleration) is set as 20*Max acceleration */
delay = 3;       %output trajectory is set as zero in the peroid of delay */
freq  = 1.0/ts;    %sampling frequency/
pause =1;		%when the trajectory moves to zero position and final position, pause 1 sec */


% compute initial condition of each trajectory segment */
t0  = pause;
t1  = a_M/j_M; %加速度增大
t2  = v_M/a_M - a_M/j_M;%加速度不变
t3  = a_M/j_M;

a1 = j_M*t1;
a2 = a1;
a3 = a2 - j_M*t3;

v1 = j_M*t1*t1/2.0;
v2 = v1 + a1*t2;
v3 = v2 + a2*t3 - j_M*t3*t3/2.0;

s1 = j_M*t1*t1*t1/6;
s2 = s1 + v1*t2 + a1*t2*t2/2.0;
s3 = s2 + v2*t3 + a2*t3*t3/2.0 - j_M*t3*t3*t3/6.0;

t4  = (p_end - 2.0*s3)/v_M;
t5  = a_M/j_M;
t6  = v_M/a_M - a_M/j_M;
t7  = a_M/j_M;
t8  = pause;
t9  = pause;
t10 = a_M/j_M;
t11 = v_M/a_M - a_M/j_M;
t12 = a_M/j_M;
t13 = (p_end - 2.0*s3)/v_M;
t14 = a_M/j_M;
t15 = v_M/a_M - a_M/j_M;
t16 = a_M/j_M;
t17 = pause;

a4  = a3;
a5  = a4 - j_M*t5;
a6  = a5;
a7  = a6 + j_M*t7;
a8  = a7;
a9  = a8;
a10 = a9 - j_M*t10;
a11 = a10;
a12 = a11 + j_M*t12;
a13 = a12;
a14 = a13 + j_M*t14;
a15 = a14;

v4  = v3 + a3*t4;
v5  = v4 + a4*t5 - j_M*t5*t5/2.0;
v6  = v5 + a5*t6;
v7  = v6 + a6*t7 + j_M*t7*t7/2.0;
v8  = v7 + a7*t8;
v9  = v8 + a8*t9;
v10 = v9 + a9*t10 - j_M*t10*t10/2.0;
v11 = v10 + a10*t11;
v12 = v11 + a11*t12 + j_M*t12*t12/2.0;
v13 = v12 + a12*t13;
v14 = v13 + a13*t14 + j_M*t14*t14/2.0;
v15 = v14 + a14*t15;

s4  = s3 + v3*t4 + a3*t4*t4/2.0;
s5  = s4 + v4*t5 + a4*t5*t5/2.0 - j_M*t5*t5*t5/6.0;
s6  = s5 + v5*t6 + a5*t6*t6/2.0;
s7  = s6 + v6*t7 + a6*t7*t7/2.0 + j_M*t7*t7*t7/6.0;
s8  = s7 + v7*t8 + a7*t8*t8/2.0;
s9  = s8 + v8*t9 + a8*t9*t9/2.0;
s10 = s9 + v9*t10 + a9*t10*t10/2.0 - j_M*t10*t10*t10/6.0;
s11 = s10 + v10*t11 + a10*t11*t11/2.0;
s12 = s11 + v11*t12 + a11*t12*t12/2.0 + j_M*t12*t12*t12/6.0;
s13 = s12 + v12*t13 + a12*t13*t13/2.0;
s14 = s13 + v13*t14 + a13*t14*t14/2.0 + j_M*t14*t14*t14/6.0;
s15 = s14 + v14*t15 + a14*t15*t15/2.0;
s16 = s15 + v15*t16 + a15*t16*t16/2.0 - j_M*t16*t16*t16/6.0;

T0  = t0;
T1  = T0 + t1;
T2  = T1 + t2;
T3  = T2 + t3;
T4  = T3 + t4;
T5  = T4 + t5;
T6  = T5 + t6;
T7  = T6 + t7;
T8  = T7 + t8;
T9  = T8 + t9;
T10 = T9 + t10;
T11 = T10 + t11;
T12 = T11 + t12;
T13 = T12 + t13;
T14 = T13 + t14;
T15 = T14 + t15;
T16 = T15 + t16;
T17 = T16 + t17;

%/* generate trajectory */
if(t<=delay)
    y(4) = 0.0;	   % /* jerk */
    y(2) = 0.0;		%/* acceleration */
    y(3) = 0.0;		%/* velocity */
    y(1) = 0.0;		%/* position */
else
    % 	 q0	  = *uPtrs[0];%q0 is what?
    T	  = T17*freq;
    tt   = (t-delay)*freq;
    rt   = mod(tt,T);
    rrt  = rt/freq;
    
    if(rt<=T0*freq)
        y(4) = 0.0;	   % /* jerk */
        y(3) = 0.0;		%/* acceleration */
        y(2) = 0.0;		%/* velocity */
        y(1) = 0.0;		%/* position */
    end
    
    if(rt>T0*freq && rt<=T1*freq)
        y(4) = j_M;
        y(3) = j_M*(rrt-T0);
        y(2) = j_M*(rrt-T0)*(rrt-T0)/2.0;
        y(1) = j_M*(rrt-T0)*(rrt-T0)*(rrt-T0)/6.0;
    end
    
    
    if(rt>T1*freq && rt<=T2*freq)
        y(4) = 0.0;
        y(3) = a1;
        y(2) = v1 + a1*(rrt-T1);
        y(1) = s1 + v1*(rrt-T1) + a1*(rrt-T1)*(rrt-T1)/2.0;
    end
    
    
    if(rt>T2*freq && rt<=T3*freq)
        y(4) = -j_M;
        y(3) = a2 - j_M*(rrt-T2);
        y(2) = v2 + a2*(rrt-T2) - j_M*(rrt-T2)*(rrt-T2)/2.0;
        y(1) = s2 + v2*(rrt-T2) + a2*(rrt-T2)*(rrt-T2)/2.0 - j_M*(rrt-T2)*(rrt-T2)*(rrt-T2)/6.0;
    end
    
    
    if(rt>T3*freq && rt<=T4*freq)
        y(4) = 0.0;
        y(3) = a3;
        y(2) = v3 + a3*(rrt-T3);
        y(1) = s3 + v3*(rrt-T3) + a3*(rrt-T3)*(rrt-T3)/2.0;
    end
    
    
    if(rt>T4*freq && rt<=T5*freq)
        y(4) = -j_M;
        y(3) = a4 - j_M*(rrt-T4);
        y(2) = v4 + a4*(rrt-T4) - j_M*(rrt-T4)*(rrt-T4)/2.0;
        y(1) = s4 + v4*(rrt-T4) + a4*(rrt-T4)*(rrt-T4)/2.0 - j_M*(rrt-T4)*(rrt-T4)*(rrt-T4)/6.0;
    end
    
    
    if(rt>T5*freq && rt<=T6*freq)
        y(4) = 0;
        y(3) = a5;
        y(2) = v5 + a5*(rrt-T5);
        y(1) = s5 + v5*(rrt-T5) + a5*(rrt-T5)*(rrt-T5)/2.0;
    end
    
    
    if(rt>T6*freq && rt<=T7*freq)
        y(4) = j_M;
        y(3) = a6 + j_M*(rrt-T6);
        y(2) = v6 + a6*(rrt-T6) + j_M*(rrt-T6)*(rrt-T6)/2.0;
        y(1) = s6 + v6*(rrt-T6) + a6*(rrt-T6)*(rrt-T6)/2.0 + j_M*(rrt-T6)*(rrt-T6)*(rrt-T6)/6.0;
    end
    
    
    if(rt>T7*freq && rt<=T8*freq)
        y(4) = 0.0;
        y(3) = 0.0;
        y(2) = 0.0;
        y(1) = s7;
    end
    
    
    if(rt>T8*freq && rt<=T9*freq)
        y(4) = 0.0;
        y(3) = 0.0;
        y(2) = 0.0;
        y(1) = s8;
    end
    
    
    if(rt>T9*freq && rt<=T10*freq)
        y(4) = -j_M;
        y(3) = a9 - j_M*(rrt-T9);
        y(2) = v9 + a9*(rrt-T9) - j_M*(rrt-T9)*(rrt-T9)/2.0;
        y(1) = s9 + v9*(rrt-T9) + a9*(rrt-T9)*(rrt-T9)/2.0 - j_M*(rrt-T9)*(rrt-T9)*(rrt-T9)/6.0;
    end
    
    
    if(rt>T10*freq && rt<=T11*freq)
        y(4) = 0.0;
        y(3) = a10;
        y(2) = v10 + a10*(rrt-T10);
        y(1) = s10 + v10*(rrt-T10) + a10*(rrt-T10)*(rrt-T10)/2.0;
    end
    
    
    
    if(rt>T11*freq && rt<=T12*freq)
        y(4) = j_M;
        y(3) = a11 + j_M*(rrt-T11);
        y(2) = v11 + a11*(rrt-T11) + j_M*(rrt-T11)*(rrt-T11)/2.0;
        y(1) = s11 + v11*(rrt-T11) + a11*(rrt-T11)*(rrt-T11)/2.0 + j_M*(rrt-T11)*(rrt-T11)*(rrt-T11)/6.0;
    end
    
    
    if(rt>T12*freq && rt<=T13*freq)
        y(4) = 0;
        y(3) = a12;
        y(2) = v12 + a12*(rrt-T12);
        y(1) = s12 + v12*(rrt-T12) + a12*(rrt-T12)*(rrt-T12)/2.0;
    end
    
    
    if(rt>T13*freq && rt<=T14*freq)
        y(4) = j_M;
        y(3) = a13 + j_M*(rrt-T13);
        y(2) = v13 + a13*(rrt-T13) + j_M*(rrt-T13)*(rrt-T13)/2.0;
        y(1) = s13 + v13*(rrt-T13) + a13*(rrt-T13)*(rrt-T13)/2.0 + j_M*(rrt-T13)*(rrt-T13)*(rrt-T13)/6.0;
    end
    
    
    if(rt>T14*freq && rt<=T15*freq)
        y(4) = 0.0;
        y(3) = a14;
        y(2) = v14 + a14*(rrt-T14);
        y(1) = s14 + v14*(rrt-T14) + a14*(rrt-T14)*(rrt-T14)/2.0;
    end
    
    
    if(rt>T15*freq && rt<=T16*freq)
        y(4) = -j_M;
        y(3) = a15 - j_M*(rrt-T15);
        y(2) = v15 + a15*(rrt-T15) - j_M*(rrt-T15)*(rrt-T15)/2.0;
        y(1) = s15 + v15*(rrt-T15) + a15*(rrt-T15)*(rrt-T15)/2.0 - j_M*(rrt-T15)*(rrt-T15)*(rrt-T15)/6.0;
    end
    
    
    if(rt>T16*freq && rt<=T17*freq)
        y(4) = 0.0;
        y(3) = 0.0;
        y(2) = 0.0;
        y(1) = s16;
    end
end
s = y(1);
v = y(2);
a = y(3);
j = y(4);

== matlab function RBFNN_1221/limit_u1 ==
  data: u input; y output
function y = fcn(u)
y=u;
if u>10
    y=10;
end
if u<-10
    y=-10;
end
end

== matlab function RBFNN_1221/Angle from IMU/MATLAB Function1 ==
  data: u input; y output
% function y = fcn(u)
% x=u;
% if x > 0.9
%     y = 0;
% else
% y = 450*(0.9-x);
% end
function y = fcn(u)
y=[0;0;0;0];
x=u;
for i = 1:4
if x(i) < 1
    y(i) = 0;
else
y(i) = 45*(x(i)-1);
end
end
end
